simulink model "traffic_actuated_signal"  (R2022b)
settings: Solver=ode1  StartTime=0.0  StopTime=inf  FixedStep=0.001  RelTol=1e-3
libraries: simulink x1
settings Model: Creator=user  LastModifiedBy=user

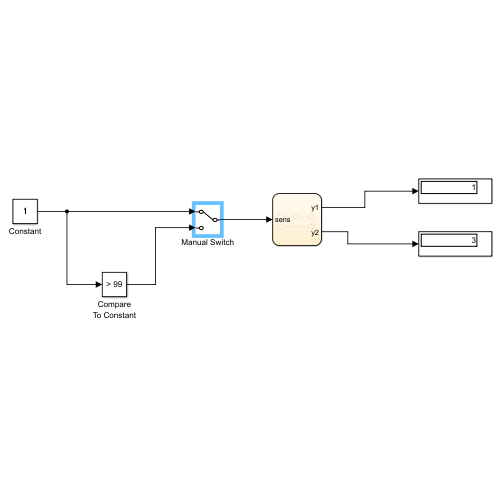
[thumbnail: Simulink's stored preview of the top-level diagram]
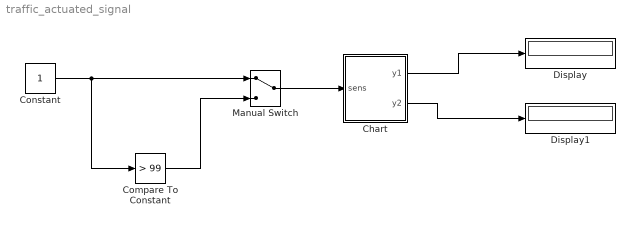
== system traffic_actuated_signal ==
  Chart : Stateflow chart  TreatAsAtomicUnit=on
  Compare To Constant : simulink/Logic and Bit Operations/Compare To Constant  relop=>  const=99  OutDataTypeStr=boolean
  Constant : Constant
  Display : Display
  Display1 : Display
  Manual Switch : ManualSwitch
  wires:
  Constant/1 -> Compare To Constant/1, Manual Switch/1
  Compare To Constant/1 -> Manual Switch/2
  Manual Switch/1 -> Chart/1(sens)
  Chart/2(y2) -> Display1/1
  Chart/1(y1) -> Display/1

== stateflow chart traffic_actuated_signal/Chart ==
  settings: executeAtInitialization=1
  state Stop
    y1 = RED;
    y2 = GREEN;
  state StopForTraffic
    y1 = RED;
    y2 = GREEN;
  state StopToGo
    y1 = RED;
    y2 = YELLOW;
  state Stop4
    y1 = YELLOW;
    y2 = RED;
  state Stop3
    y1 = GREEN;
    y2 = RED;
  (default) -> Stop
  StopForTraffic -> StopToGo : [sens]
  Stop -> StopForTraffic : after(20, sec)
  Stop4 -> Stop : after(3, sec)
  StopToGo -> Stop3 : after(3, sec)
  Stop3 -> Stop4 : after(10, sec)
  data: RED constant double =1; YELLOW constant double =2; GREEN constant double =3; sens input; y1 output; y2 output
